simulink model "q3"  (R2021b)
settings: Solver=VariableStepAuto  StartTime=0.0  StopTime=10.0  RelTol=1e-3
settings Model: Creator=alimi  LastModifiedBy=alimi

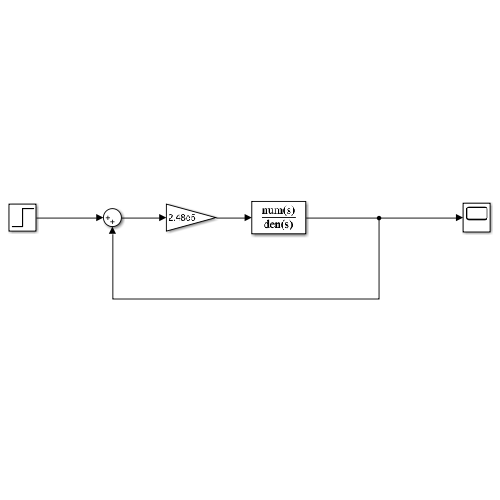
[thumbnail: Simulink's stored preview of the top-level diagram]
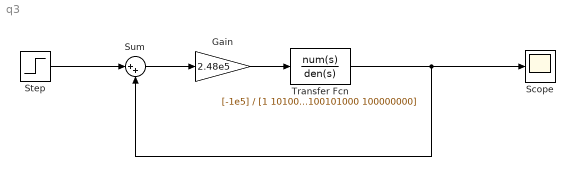
== system q3 ==
  Gain : Gain  Gain=2.48e5
  Scope : Scope
  Step : Step  Time=0.000000001  SampleTime=0
  Sum : Sum  Inputs=|++
  Transfer Fcn : TransferFcn  Numerator=[-1e5]  Denominator=[1 101001 100101000 100000000]
  wires:
  Gain/1 -> Transfer Fcn/1
  Transfer Fcn/1 -> Sum/2, Scope/1
  Sum/1 -> Gain/1
  Step/1 -> Sum/1
